simulink subsystem "canInputs"  (R2023b)
settings: Solver=VariableStepAuto  StartTime=0.0  StopTime=10.0  RelTol=1e-3
libraries: Raptor_lib x2, canmsglib x1
settings Model: Creator=serga  LastModifiedBy=serga
settings OptimizationCC: ReuseModelBlockBuffer=off

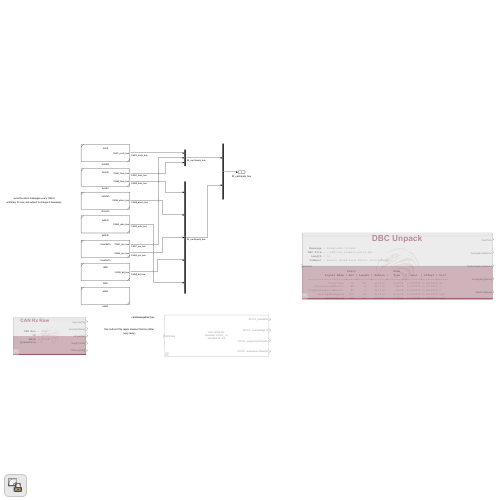
[thumbnail: Simulink's stored preview of the top-level diagram]
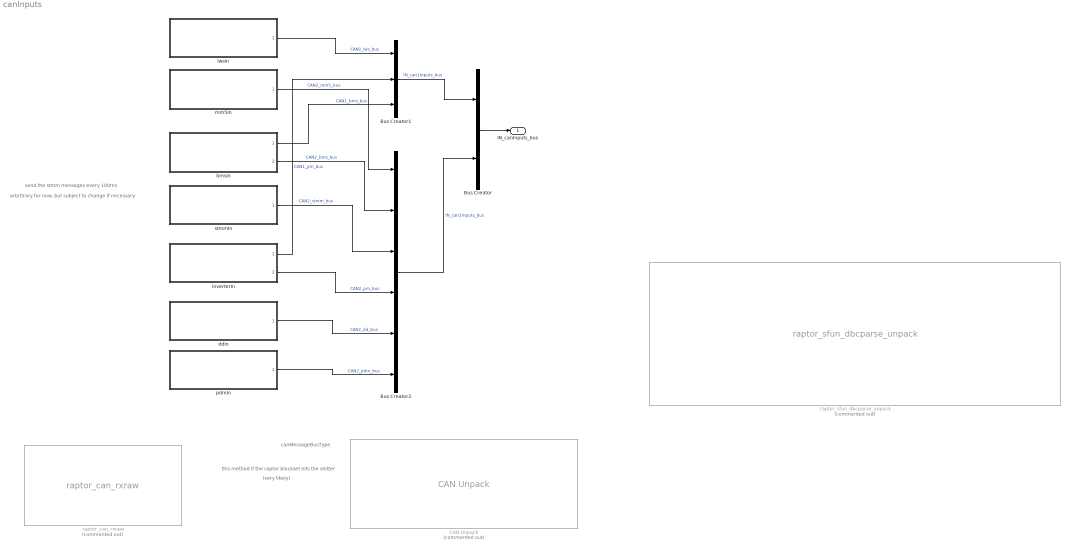
== system canInputs ==
  note: (very likely)
  note: this method if the raptor blockset hits the shitter
  note: arbritrary for now, but subject to change if necessary
  note: send the stmm messages every 100ms
  note: canMessageBusType
  Bus Creator : BusCreator  Inputs=2
  Bus Creator1 : BusCreator  Inputs=3
  Bus Creator2 : BusCreator  Inputs=6
  CAN Unpack : canmsglib/CAN Unpack  Commented=on  CANdbFile=C:\eagle_EVSR24\CAN\redacted\CAN2.dbc  MsgList=ATCCF_10  MsgName=ATCCF_10  MsgIDType=Standard (11-bit identifier)  MsgIdentifier=410  MsgLength=8  SignalInfo={'ATCCF_brakeBias','16','16','LE','signed','Standard','0','0.1','0','0','100';'ATCCF_counterMsg410','0','4','LE','unsigned','Standard','0','1','0','0','15';'ATCCF_suspensionTravelFL','32','16','LE','signed','Standard','0','0.001','0','-32.768','32.767';'ATCCF_suspensionTravelFR','48','16','LE','signed','Standard','0','0.001','0','-32.768','32.767'}  IDPort=off  TimestampPort=off  ErrorPort=off  RemotePort=off  LengthPort=off  StatusPort=off  ApplyMinMax=off
      settings: LibrarySourceBlock=embeddedtargetslib/Host Communication/CAN Unpack  DataFormat=CANdb specified signals
  bmsIn : Subsystem  ReferencedSubsystem=bmsIn
  ddIn : Subsystem  ReferencedSubsystem=ddIn
  inverterIn : Subsystem  ReferencedSubsystem=inverterIn
  lwsIn : Subsystem  ReferencedSubsystem=lwsIn
  mm5In : Subsystem  ReferencedSubsystem=mm5In
  pdmIn : Subsystem  ReferencedSubsystem=pdmIn
  raptor_can_rxraw : Raptor_lib/CAN/raptor_can_rxraw  Commented=on  canBus='CAN1'  extendedId=0  showAge=1  id=hex2dec('100')  idMask=hex2dec('1FFFFFFF')  mailbox=''  queueSize=1  useSimFunc=0  sim_func_name=''  create_btn=[]  update_btn=[]
      settings: SourceProductName=Raptor
  raptor_sfun_dbcparse_unpack : Raptor_lib/CAN/raptor_sfun_dbcparse_unpack  Commented=on  message=struct('name', 'ExampleMulttFrame', 'description' , 'Engine Speed/Load Factor Information', 'payload_size', 16, 'SignalInfo', {{struct('Name', 'TotalTime', 'description', 'Total time.', 'StartBit', 48, 'SignalSize', 32, 'ByteOrder' , 'LittleEndian', 'ValueType' , 'Integer', 'Class', 'uint32', 'Signed', '0', 'Factor', 0.05, 'Offset', 0, 'Min', 0, 'Max', 0, 'Units', 'hr', 'Comment', 'Total time.'), struct('Name', 'AverageLoadFactor', 'description', 'Average engine load factor ', 'StartBit', 40, 'SignalSize', 8, 'ByteOrder' , 'LittleEndian', 'ValueType' , 'Integer', 'Class', 'uint8', 'Signed', '0', 'Factor', 0.4, 'Offset', 0, 'Min', 0, 'Max', 0, 'Units', '%', 'Comment', 'Average engine load factor '), struct('Name', 'TripAverageLoadFactor', 'description', 'Average engine load factor for current trip.', 'StartBit', 32, 'SignalSize', 8, 'ByteOrder' , 'LittleEndian', 'ValueType' , 'Integer', 'Class', 'uint8', 'Signed', '0', 'Factor', 0.4, 'Offset', 0, 'Min', 0, 'Max', 0, 'Units', '%', 'Comment', 'Average engine load factor for current trip.'), struct('Name', 'AverageEngSpeed', 'description', 'Average speed of the engine since the last trip reset.', 'StartBit', 16, 'SignalSize', 16, 'ByteOrder' , 'LittleEndian', 'ValueType' , 'Integer', 'Class', 'uint16', 'Signed', '0', 'Factor', 0.125, 'Offset', 0, 'Min', 0, 'Max', 0, 'Units', 'rpm', 'Comment', 'Average speed of the engine since the last trip reset.'), struct('Name', 'MaxEngSpeed', 'description', 'Maximum engine speed achieved since the last trip reset.', 'StartBit', 0, 'SignalSize', 16, 'ByteOrder' , 'LittleEndian', 'ValueType' , 'Integer', 'Class', 'uint16', 'Signed', '0', 'Factor', 0.125, 'Offset', 0, 'Min', 0, 'Max', 0, 'Units', 'rpm', 'Comment', 'Maximum engine speed achieved since the last trip reset.')}})  settings=struct('File','.\CAN\can_example_multi.dbc','SelectedMessage','ExampleMulttFrame','UnassignedBits','','LabelWire','on','ShowRaw','off','signalOrder','0','EnabledSignals', {{'TotalTime','AverageLoadFactor','TripAverageLoadFactor','AverageEngSpeed','MaxEngSpeed',}})
      settings: SourceProductName=Raptor
  stmmIn : Subsystem  ReferencedSubsystem=stmmIn
  IN_canInputs_bus : Outport
  wires:
  Bus Creator/1 -> IN_canInputs_bus/1
  mm5In/1 -> Bus Creator2/1  "CAN2_mm5_bus"
  Bus Creator1/1 -> Bus Creator/1  "IN_can1Inputs_bus"
  stmmIn/1 -> Bus Creator2/3  "CAN2_stmm_bus"
  Bus Creator2/1 -> Bus Creator/2  "IN_can2Inputs_bus"
  inverterIn/2 -> Bus Creator2/4  "CAN2_pm_bus"
  inverterIn/1 -> Bus Creator1/2  "CAN1_pm_bus"
  ddIn/1 -> Bus Creator2/5  "CAN2_dd_bus"
  bmsIn/1 -> Bus Creator1/3  "CAN1_bms_bus"
  bmsIn/2 -> Bus Creator2/2  "CAN2_bms_bus"
  pdmIn/1 -> Bus Creator2/6  "CAN2_pdm_bus"
  lwsIn/1 -> Bus Creator1/1  "CAN1_lws_bus"
